simulink model "PIDcoaxial"  (Simulink 6.6)
settings: Solver=ode45  StartTime=0.0  StopTime=10.0  MaxStep=0.5  MinStep=0.1  RelTol=1e-3
values from neighbouring files (symbols this model uses):
  hdreq = in_states(7)    [RunfileCoaxialDynamic.m]    (also in Runfile_maxquickness.m)
  in_controls = controls(N,:)'    [Maxpitchquicknessoutput.m]    (also in Pitchquicknessoutput.m; Rollquicknessoutput.m; RunfileCoaxialDynamic.m; Runfile_maxquickness.m)
  in_states = states(N,:)'    [Maxpitchquicknessoutput.m]    (also in Pitchquicknessoutput.m; Rollquicknessoutput.m; RunfileCoaxialDynamic.m; Runfile_maxquickness.m)
  Kdiffl = 0.5    [RunfileCoaxialDynamic.m]    (also in Runfile_maxquickness.m)
  Kdiffu = 0.5    [RunfileCoaxialDynamic.m]    (also in Runfile_maxquickness.m)
  Kp = -0.3    [RunfileCoaxialDynamic.m]    (also in Runfile_maxquickness.m = -0.2)
  Kphi = 0.4    [RunfileCoaxialDynamic.m]    (also in Runfile_maxquickness.m = 0.6)
  Kphi_int = 0.002    [RunfileCoaxialDynamic.m]    (also in Runfile_maxquickness.m = -0.02)
  Kpsi = 0.7    [RunfileCoaxialDynamic.m]    (also in Runfile_maxquickness.m)
  Kpsi_int = -0.001    [RunfileCoaxialDynamic.m]    (also in Runfile_maxquickness.m)
  Kq = 0.3    [RunfileCoaxialDynamic.m]    (also in Runfile_maxquickness.m = 0.6)
  Kr = -0.4    [RunfileCoaxialDynamic.m]    (also in Runfile_maxquickness.m)
  Ktheta = -0.8    [RunfileCoaxialDynamic.m]    (also in Runfile_maxquickness.m = -3.1)
  Ktheta_int = -0.1    [RunfileCoaxialDynamic.m]    (also in Runfile_maxquickness.m)
  Kz = -0.005    [RunfileCoaxialDynamic.m]    (also in Runfile_maxquickness.m)
  Kz_int = 0    [RunfileCoaxialDynamic.m]    (also in Runfile_maxquickness.m)
  Kzdot = 0    [RunfileCoaxialDynamic.m]    (also in Runfile_maxquickness.m)
  phiFreq = in_states(9)    [RunfileCoaxialDynamic.m]    (also in Runfile_maxquickness.m)
  t_hd = 0    [RunfileCoaxialDynamic.m]    (also in Runfile_maxquickness.m)
  t_phi = 0    [RunfileCoaxialDynamic.m]    (also in Runfile_maxquickness.m)
  t_theta = 0    [RunfileCoaxialDynamic.m]    (also in Runfile_maxquickness.m = 0.2)
  t_z = 0    [RunfileCoaxialDynamic.m]    (also in Runfile_maxquickness.m)
  thetaFreq = in_states(8)    [RunfileCoaxialDynamic.m]    (also in Runfile_maxquickness.m = 30*pi/180+in_states(8))
  xInitial = [in_states]    [RunfileCoaxialDynamic.m]    (also in Runfile_maxquickness.m)
  zreq = -hreq    [RunfileCoaxialDynamic.m]    (also in Runfile_maxquickness.m)
settings Model: Creator=John  LastModifiedBy=John
settings DebuggingCC: SignalResolutionControl=TryResolveAllWithWarning  MultiTaskDSMMsg=warning  MultiTaskCondExecSysMsg=none
settings RTWCC: IncludeERTFirstTime=on

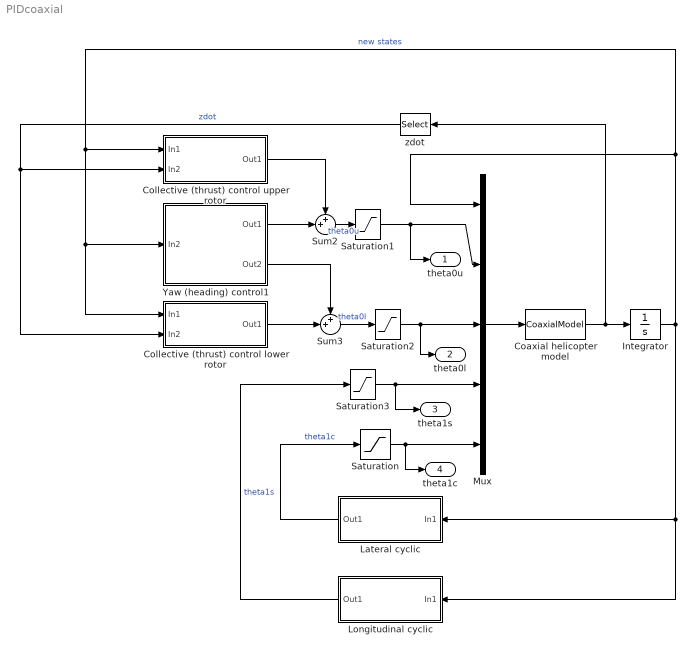
== system PIDcoaxial ==
  Coaxial helicopter model : MATLABFcn  MATLABFcn=CoaxialModel  OutputDimensions=14
  Collective (thrust) control lower rotor : Subsystem
  Collective (thrust) control upper rotor : Subsystem
  Integrator : Integrator  InitialCondition=xInitial
  Lateral cyclic : Subsystem  Orientation=left
  Longitudinal cyclic : Subsystem  Orientation=left
  Mux : Mux  Inputs=5
  Saturation : Saturate  UpperLimit=6.75*pi/180  LowerLimit=-6.75*pi/180
  Saturation1 : Saturate  UpperLimit=25*pi/180  LowerLimit=0
  Saturation2 : Saturate  UpperLimit=25*pi/180  LowerLimit=0
  Saturation3 : Saturate  UpperLimit=15*pi/180  LowerLimit=-15*pi/180
  Sum2 : Sum  Inputs=++|
  Sum3 : Sum  Inputs=++|
  Yaw (heading) control1 : Subsystem
  zdot : Selector  Orientation=left  IndexOptions=Index vector (dialog)  Indices=[12]  OutputSizes=1  InputPortWidth=14
  theta0u : Outport
  theta0l : Outport  Port=2
  theta1s : Outport  Port=3
  theta1c : Outport  Port=4
  wires:
  Coaxial helicopter model/1 -> Integrator/1, zdot/1
  Integrator/1 -> Mux/1, Collective (thrust) control upper rotor/1(In1), Collective (thrust) control lower rotor/1(In1), Yaw (heading) control1/1(In2), Longitudinal cyclic/1(In1), Lateral cyclic/1(In1)  "new states"
  Mux/1 -> Coaxial helicopter model/1
  Lateral cyclic/1(Out1) -> Saturation/1  "theta1c"
  Yaw (heading) control1/2(Out2) -> Sum3/1
  zdot/1 -> Collective (thrust) control lower rotor/2(In2), Collective (thrust) control upper rotor/2(In2)  "zdot"
  Yaw (heading) control1/1(Out1) -> Sum2/2
  Sum2/1 -> Saturation1/1  "theta0u"
  Collective (thrust) control upper rotor/1(Out1) -> Sum2/1
  Collective (thrust) control lower rotor/1(Out1) -> Sum3/2
  Sum3/1 -> Saturation2/1  "theta0l"
  Longitudinal cyclic/1(Out1) -> Saturation3/1  "theta1s"
  Saturation/1 -> Mux/5, theta1c/1
  Saturation1/1 -> Mux/2, theta0u/1
  Saturation2/1 -> Mux/3, theta0l/1
  Saturation3/1 -> Mux/4, theta1s/1

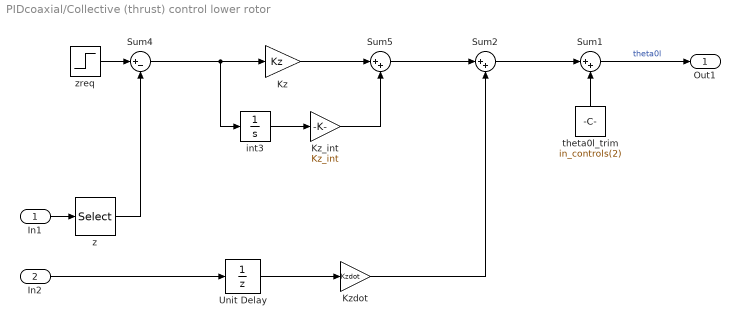
== system PIDcoaxial/Collective (thrust) control lower rotor ==
  In1 : Inport
  In2 : Inport  Port=2
  Kz : Gain  Gain=Kz
  Kz_int : Gain  Gain=Kz_int
  Kzdot : Gain  Gain=Kzdot
  Sum1 : Sum  Inputs=|++  SaturateOnIntegerOverflow=on
  Sum2 : Sum  Inputs=|++  SaturateOnIntegerOverflow=on
  Sum4 : Sum  Inputs=|+-  SaturateOnIntegerOverflow=on
  Sum5 : Sum  Inputs=|++  SaturateOnIntegerOverflow=on
  Unit Delay : UnitDelay
  int3 : Integrator
  theta0l_trim : Constant  Orientation=up  Value=in_controls(2)
  z : Selector  IndexOptions=Index vector (dialog)  Indices=[12]  OutputSizes=1  InputPortWidth=14
  zreq : Step  Time=t_z  Before=in_states(12)  After=zreq  SampleTime=0
  Out1 : Outport
  wires:
  zreq/1 -> Sum4/1
  int3/1 -> Kz_int/1
  theta0l_trim/1 -> Sum1/2
  Sum1/1 -> Out1/1  "theta0l"
  Sum4/1 -> Kz/1, int3/1
  Kz/1 -> Sum5/1
  Kz_int/1 -> Sum5/2
  In2/1 -> Unit Delay/1
  Unit Delay/1 -> Kzdot/1
  Kzdot/1 -> Sum2/2
  Sum2/1 -> Sum1/1
  Sum5/1 -> Sum2/1
  In1/1 -> z/1
  z/1 -> Sum4/2

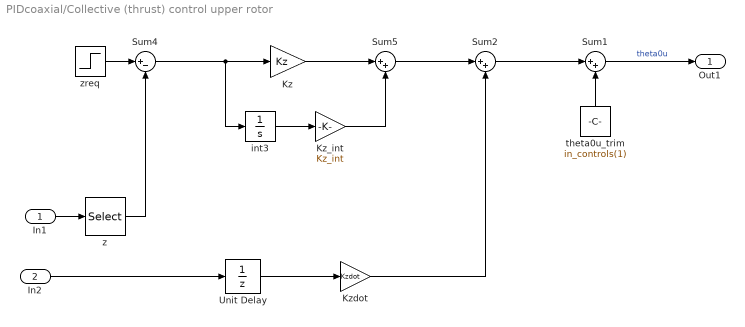
== system PIDcoaxial/Collective (thrust) control upper rotor ==
  In1 : Inport
  In2 : Inport  Port=2
  Kz : Gain  Gain=Kz
  Kz_int : Gain  Gain=Kz_int
  Kzdot : Gain  Gain=Kzdot
  Sum1 : Sum  Inputs=|++  SaturateOnIntegerOverflow=on
  Sum2 : Sum  Inputs=|++  SaturateOnIntegerOverflow=on
  Sum4 : Sum  Inputs=|+-  SaturateOnIntegerOverflow=on
  Sum5 : Sum  Inputs=|++  SaturateOnIntegerOverflow=on
  Unit Delay : UnitDelay
  int3 : Integrator
  theta0u_trim : Constant  Orientation=up  Value=in_controls(1)
  z : Selector  IndexOptions=Index vector (dialog)  Indices=[12]  OutputSizes=1  InputPortWidth=14
  zreq : Step  Time=t_z  Before=in_states(12)  After=zreq  SampleTime=0
  Out1 : Outport
  wires:
  zreq/1 -> Sum4/1
  int3/1 -> Kz_int/1
  Sum4/1 -> Kz/1, int3/1
  Kz/1 -> Sum5/1
  Kz_int/1 -> Sum5/2
  In2/1 -> Unit Delay/1
  Unit Delay/1 -> Kzdot/1
  Sum5/1 -> Sum2/1
  Sum2/1 -> Sum1/1
  Kzdot/1 -> Sum2/2
  In1/1 -> z/1
  Sum1/1 -> Out1/1  "theta0u"
  theta0u_trim/1 -> Sum1/2
  z/1 -> Sum4/2

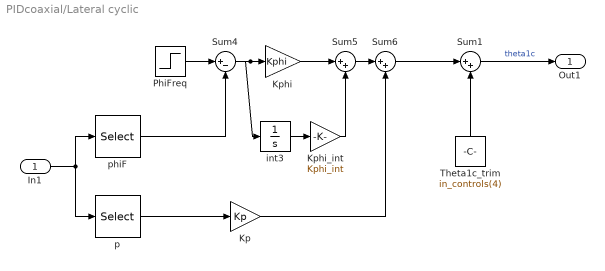
== system PIDcoaxial/Lateral cyclic ==
  In1 : Inport
  Kp : Gain  Gain=Kp
  Kphi : Gain  Gain=Kphi
  Kphi_int : Gain  Gain=Kphi_int
  PhiFreq : Step  Time=t_phi  Before=in_states(9)  After=phiFreq  SampleTime=0
  Sum1 : Sum  Inputs=|++  SaturateOnIntegerOverflow=on
  Sum4 : Sum  Inputs=|+-  SaturateOnIntegerOverflow=on
  Sum5 : Sum  Inputs=|++  SaturateOnIntegerOverflow=on
  Sum6 : Sum  Inputs=|++  SaturateOnIntegerOverflow=on
  Theta1c_trim : Constant  Orientation=up  Value=in_controls(4)
  int3 : Integrator
  p : Selector  IndexOptions=Index vector (dialog)  Indices=[4]  OutputSizes=1  InputPortWidth=14
  phiF : Selector  IndexOptions=Index vector (dialog)  Indices=[9]  OutputSizes=1  InputPortWidth=14
  Out1 : Outport
  wires:
  p/1 -> Kp/1
  In1/1 -> phiF/1, p/1
  PhiFreq/1 -> Sum4/1
  int3/1 -> Kphi_int/1
  Kphi_int/1 -> Sum5/2
  Kphi/1 -> Sum5/1
  Sum4/1 -> Kphi/1, int3/1
  Sum5/1 -> Sum6/1
  phiF/1 -> Sum4/2
  Kp/1 -> Sum6/2
  Sum6/1 -> Sum1/1
  Sum1/1 -> Out1/1  "theta1c"
  Theta1c_trim/1 -> Sum1/2

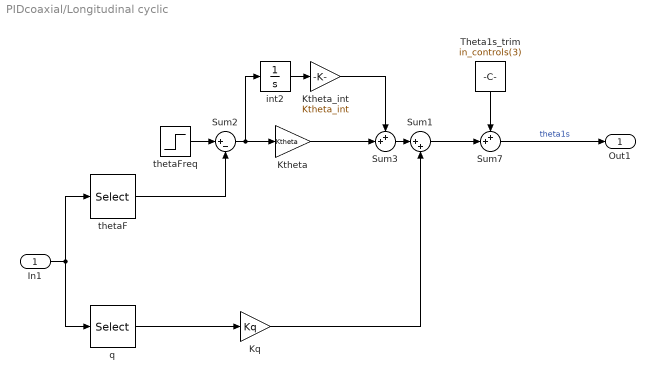
== system PIDcoaxial/Longitudinal cyclic ==
  In1 : Inport
  Kq : Gain  Gain=Kq
  Ktheta : Gain  Gain=Ktheta
  Ktheta_int : Gain  Gain=Ktheta_int
  Sum1 : Sum  Inputs=|++  SaturateOnIntegerOverflow=on
  Sum2 : Sum  Inputs=|+-  SaturateOnIntegerOverflow=on
  Sum3 : Sum  Inputs=++|  SaturateOnIntegerOverflow=on
  Sum7 : Sum  Inputs=++|  SaturateOnIntegerOverflow=on
  Theta1s_trim : Constant  Orientation=down  Value=in_controls(3)
  int2 : Integrator
  q : Selector  IndexOptions=Index vector (dialog)  Indices=[5]  OutputSizes=1  InputPortWidth=14
  thetaF : Selector  IndexOptions=Index vector (dialog)  Indices=[8]  OutputSizes=1  InputPortWidth=14
  thetaFreq : Step  Time=t_theta  Before=in_states(8)  After=thetaFreq  SampleTime=0
  Out1 : Outport
  wires:
  In1/1 -> thetaF/1, q/1
  Sum2/1 -> Ktheta/1, int2/1
  int2/1 -> Ktheta_int/1
  Ktheta_int/1 -> Sum3/1
  Sum3/1 -> Sum1/1
  Ktheta/1 -> Sum3/2
  thetaFreq/1 -> Sum2/1
  thetaF/1 -> Sum2/2
  q/1 -> Kq/1
  Kq/1 -> Sum1/2
  Sum1/1 -> Sum7/2
  Theta1s_trim/1 -> Sum7/1
  Sum7/1 -> Out1/1  "theta1s"

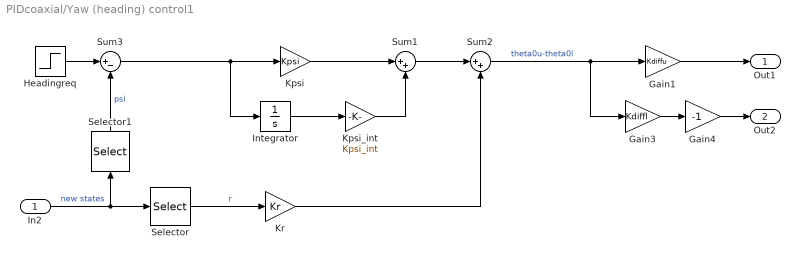
== system PIDcoaxial/Yaw (heading) control1 ==
  In2 : Inport
  Gain1 : Gain  Gain=Kdiffu
  Gain3 : Gain  Gain=Kdiffl
  Gain4 : Gain  Gain=-1
  Headingreq : Step  Time=t_hd  Before=in_states(7)  After=hdreq  SampleTime=0
  Integrator : Integrator
  Kpsi : Gain  Gain=Kpsi
  Kpsi_int : Gain  Gain=Kpsi_int
  Kr : Gain  Gain=Kr
  Selector : Selector  IndexOptions=Index vector (dialog)  Indices=[6]  OutputSizes=1  InputPortWidth=14
  Selector1 : Selector  Orientation=up  IndexOptions=Index vector (dialog)  Indices=[7]  OutputSizes=1  InputPortWidth=14
  Sum1 : Sum  Inputs=|++
  Sum2 : Sum  Inputs=|++
  Sum3 : Sum  Inputs=|+-
  Out1 : Outport
  Out2 : Outport  Port=2
  wires:
  Integrator/1 -> Kpsi_int/1
  Kpsi/1 -> Sum1/1
  Kpsi_int/1 -> Sum1/2
  Sum1/1 -> Sum2/1
  Gain4/1 -> Out2/1
  Headingreq/1 -> Sum3/1
  Sum3/1 -> Kpsi/1, Integrator/1
  In2/1 -> Selector/1, Selector1/1  "new states"
  Selector1/1 -> Sum3/2  "psi"
  Sum2/1 -> Gain1/1, Gain3/1  "theta0u-theta0l"
  Gain1/1 -> Out1/1
  Gain3/1 -> Gain4/1
  Selector/1 -> Kr/1  "r"
  Kr/1 -> Sum2/2
